simulink model "double_pendulum_dynamics"  (R2020b)
settings: Solver=VariableStepAuto  StartTime=0.0  StopTime=20  RelTol=1e-3
libraries: simulink x2
settings Model: Creator=maximilianstoelzle  LastModifiedBy=maximilianstoelzle

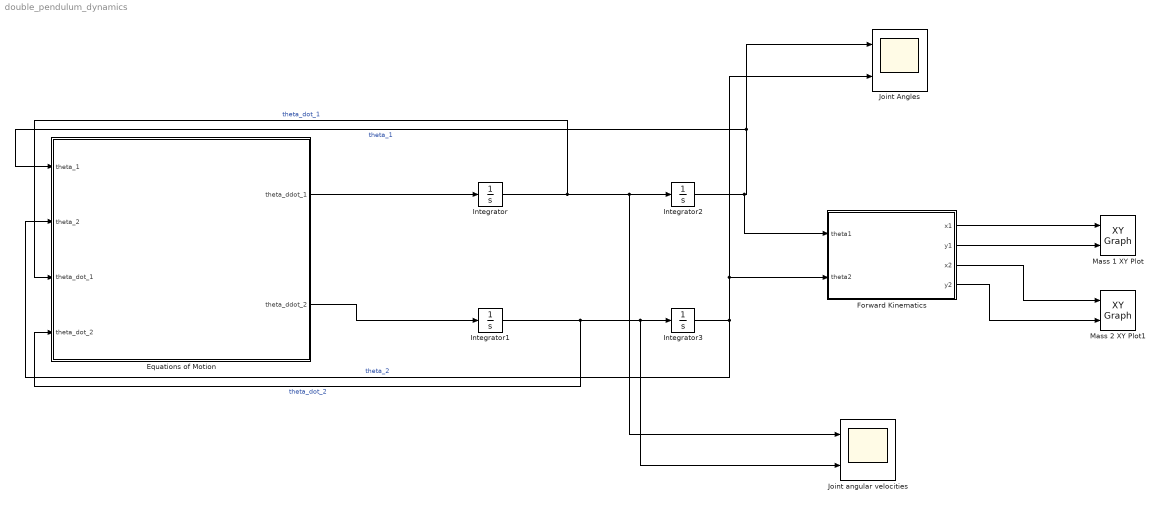
== system double_pendulum_dynamics ==
  Equations of Motion : MATLAB Function  TreatAsAtomicUnit=on
  Forward Kinematics : MATLAB Function  TreatAsAtomicUnit=on
  Integrator : Integrator
  Integrator1 : Integrator
  Integrator2 : Integrator
  Integrator3 : Integrator  InitialCondition=pi/2
  Joint Angles : Scope  NumInputPorts=2
  Joint angular velocities : Scope  NumInputPorts=2
  Mass 1 XY Plot : simulink/Sinks/XY Graph  xmin=-0.6  xmax=0.6  ymin=-0.6  ymax=0.6  st=-1
  Mass 2 XY Plot1 : simulink/Sinks/XY Graph  xmin=-1.6  xmax=1.6  ymin=-1.6  ymax=1.6  st=-1
  wires:
  Equations of Motion/1(theta_ddot_1) -> Integrator/1
  Equations of Motion/2(theta_ddot_2) -> Integrator1/1
  Integrator/1 -> Equations of Motion/3(theta_dot_1), Joint angular velocities/1, Integrator2/1  "theta_dot_1"
  Integrator1/1 -> Equations of Motion/4(theta_dot_2), Joint angular velocities/2, Integrator3/1  "theta_dot_2"
  Integrator2/1 -> Forward Kinematics/1(theta1), Equations of Motion/1(theta_1), Joint Angles/1  "theta_1"
  Integrator3/1 -> Equations of Motion/2(theta_2), Forward Kinematics/2(theta2), Joint Angles/2  "theta_2"
  Forward Kinematics/1(x1) -> Mass 1 XY Plot/1
  Forward Kinematics/2(y1) -> Mass 1 XY Plot/2
  Forward Kinematics/3(x2) -> Mass 2 XY Plot1/1
  Forward Kinematics/4(y2) -> Mass 2 XY Plot1/2

== matlab function double_pendulum_dynamics/Forward Kinematics ==
  data: theta1 input; x1 output; theta2 input; y1 output; x2 output; y2 output
function [x1, y1, x2, y2] = forward_kinematics(theta1, theta2)
    l1 = 0.5;
    l2 = 1;
    
    x1 = sin(theta1) * l1;
    y1 = -cos(theta1) * l1;
    x2 = x1 + sin(theta2) * l2;
    y2 = y1 - cos(theta2) * l2;

== matlab function double_pendulum_dynamics/Equations of Motion ==
  data: theta_1 input; theta_ddot_1 output; theta_2 input; theta_dot_1 input; theta_dot_2 input; theta_ddot_2 output
function [theta_ddot_1, theta_ddot_2]= EoM(theta_1, theta_2, theta_dot_1, theta_dot_2)
    l = 1; % [m]
    g = 9.81; % [m/s^2]
    
    M = [5/4, 1/2*cos(theta_1-theta_2); 1/2*cos(theta_1-theta_2), 1]*l;
    b = 1/2*l*sin(theta_1-theta_2)*[theta_dot_1^2; -theta_dot_2^2];
    g = g*[sin(theta_1); sin(theta_2)];
    
    % q = [theta_1; theta_2];
    % q_dot = [theta_dot_1; theta_dot_2];
    q_ddot = -pinv(M, 0.0001)*(b+g);
    theta_ddot_1 = q_ddot(1);
    theta_ddot_2 = q_ddot(2);
